simulink model "monitor_laberinto"  (R2017b)
settings: Solver=VariableStepAuto  StartTime=0.0  StopTime=inf  RelTol=1e-3
PreLoadFcn:
  | Ts=0.03;
libraries: LibrarySimulinkSAS x1, aerolibanimutils x1
settings Model: Creator=Mauro  LastModifiedBy=Mauro

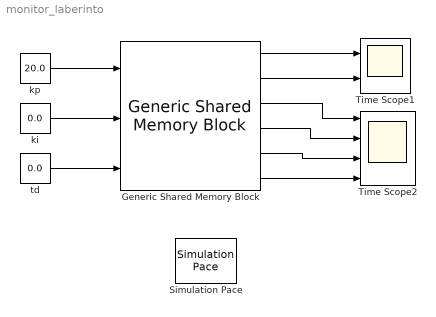
== system monitor_laberinto ==
  Generic Shared Memory Block : LibrarySimulinkSAS/Generic Shared Memory Block  nombre='ARDUINO'  dispositivo=1  vecE=[1 1 1]  vecS=[1 1 1 1 1 1]  tipoE=['f' 'f' 'f']  tipoS=['f' 'f' 'f' 'f' 'f' 'f']  ts=-1
      settings: SourceProductName=Library SAS
  Simulation Pace : aerolibanimutils/Simulation Pace  SimulationPace=1  SleepMode=MATLAB Thread  OutputPaceError=off  SampleTime=Ts/2
  Time Scope1 : Scope  NumInputPorts=2
  Time Scope2 : Scope  NumInputPorts=4
  ki : Constant  Value=0.0  OutDataTypeStr=single  SampleTime=Ts
  kp : Constant  Value=20.0  OutDataTypeStr=single  SampleTime=Ts
  td : Constant  Value=0.0  OutDataTypeStr=single  SampleTime=Ts
  wires:
  kp/1 -> Generic Shared Memory Block/1
  ki/1 -> Generic Shared Memory Block/2
  td/1 -> Generic Shared Memory Block/3
  Generic Shared Memory Block/1 -> Time Scope1/1
  Generic Shared Memory Block/2 -> Time Scope1/2
  Generic Shared Memory Block/3 -> Time Scope2/1
  Generic Shared Memory Block/4 -> Time Scope2/2
  Generic Shared Memory Block/5 -> Time Scope2/3
  Generic Shared Memory Block/6 -> Time Scope2/4
